simulink library "FInjLib"  (R2022b)
settings: Solver=VariableStepAuto  StartTime=0.0  StopTime=10.0  RelTol=1e-3
libraries: simulink x2, $bdroot x2
(part 1 of 2)
settings Model: Creator=flata  LastModifiedBy=JF
settings SolverCC: AlgebraicLoopSolver=TrustRegion
settings DebuggingCC: UnconnectedInputMsg=warning  UnconnectedOutputMsg=warning  UnconnectedLineMsg=warning  SFMachineParentedDataDiag=warning  ArithmeticOperatorsInVariantConditions=warning
settings ModelReferenceCC: EnableRefExpFcnMdlSchedulingChecks=on
settings SFSimCC: CustomCodeUndefinedFunction=UseInterfaceOnly
settings RTWCC: DLArmComputeVersion=19.05

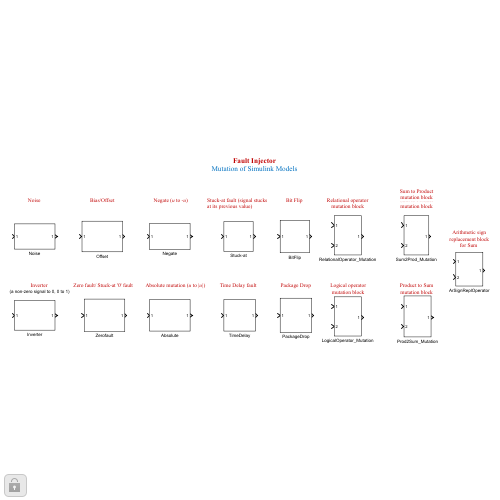
[thumbnail: Simulink's stored preview of the top-level diagram]
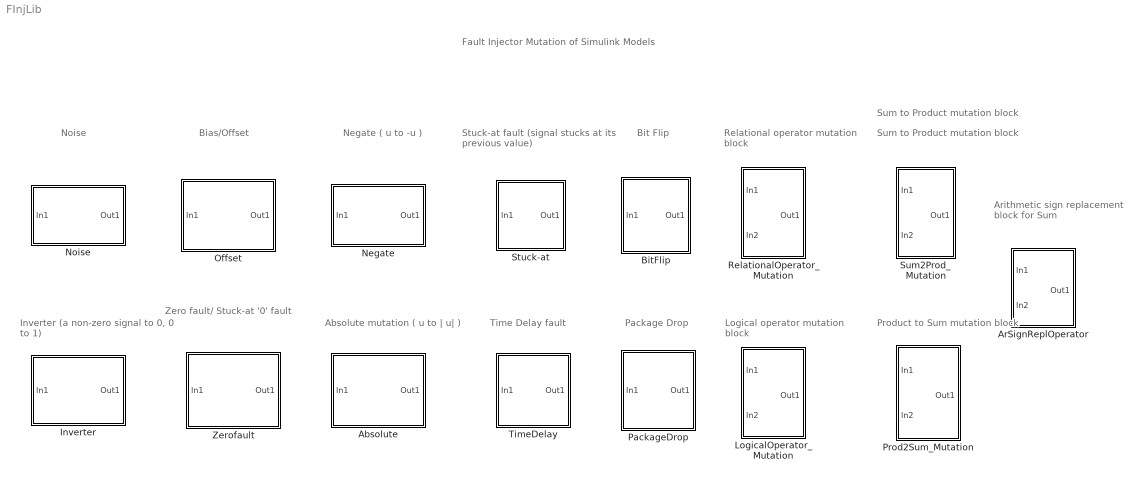
== system FInjLib ==
  note: Fault Injector
      | Mutation of Simulink Models
  note: Bias/Offset
  note: Noise
  note: Negate ( u to -u )
  note: Inverter
      | (a non-zero signal to 0, 0 to 1)
  note: Absolute mutation ( u to | u| )
  note: Zero fault/ Stuck-at '0' fault
  note: Stuck-at fault (signal stucks at its previous value)
  note: Time Delay fault
  note: Bit Flip
  note: Package Drop
  note: Relational operator mutation block
  note: Logical operator mutation block
  note: Sum to Product mutation block
  note: Product to Sum mutation block
  note: Arithmetic sign replacement block for Sum
  note: Sum to Product mutation block
  Absolute : Subsystem  mask(Absolue mutation block){FInjBlockNum=1, FIEnableflag=off, FaultOccurenceTime=0, FaultEffect=Infinite time, FaultDuration=1}
      mask prompts: FInjBlockNum "Name of the Fault Injector block"; FIEnableflag "Turn on fault injection"; FaultOccurenceTime "Enter the time of fault occurence (in seconds)"; FaultDuration "Enter the fault duration (in seconds)"
      mask help: This block makes a signal u to |u|.
      mask init:
      | a = Simulink.Mask.get(gcb);
      | Enable_signal = a.getParameter('FIEnableflag');
      | Fault_Occurence_Time = a.getParameter('FaultOccurenceTime');
      | Fault_Effect = a.getParameter('FaultEffect');
      | Fault_Duration = a.getParameter('FaultDuration');
      | 
      | value = Enable_signal.Value;
      | switch value
      |     case 'on'
      |     set_param('FInjLib/Absolute/Enable_flag', 'Value', '1');
      |     case 'off'
      |     set_param('FInjLib/Absolute/Enable_flag', 'Value', '0');
      | end
      | 
      | if Fault_Effect.Value == "Infinite time"
      |     Fault_Duration.Visible = 'off';
      | else
      |     Fault_Duration.Visible = 'on';
      | end
      | 
      | if Fault_Effect.Value == "Constant time"
      |     Fault_Duration.Prompt = "Enter the fault duration (in seconds)";
      | end
      | 
      | if Fault_Effect.Value == "Infinite time"
      |     set_param('FInjLib/Absolute/Faulttype','Value', '1');
      |     set_param('FInjLib/Absolute/Step', 'Time', Fault_Occurence_Time.Value);
      | else
      |     set_param('FInjLib/Absolute/Faulttype','Value', '2');
      |     set_param('FInjLib/Absolute/Pulse Generator', 'PhaseDelay', Fault_Occurence_Time.Value);
      |     set_param('FInjLib/Absolute/Pulse Generator', 'PulseWidth', Fault_Duration.Value);
      | end
      mask Help:
      | The block takes the following inputs:
      | - Name of the Fault Injector block ---- Feed a number as input
      | - Fault effect --- Constant time, Infinite time
      | - Fault duration --- if Fault effect is 'Constant time'
      | 
      | *For further information, see the file "README.m"
      mask TypeOptions FaultEffect: Infinite time | Constant time
      mask DialogControl Container3 Prompt: Fault Effect
  ArSignReplOperator : Subsystem  mask(Arithmetic Sign Replacement Block (for Sum)){FInjBlockNum=1, FIEnableflag=off, OperatorNum=2, FaultOccurenceTime=3, FaultEffect=Constant time, FaultDuration=5}
      mask prompts: FInjBlockNum "Name of the Fault Injector block"; FIEnableflag "Turn on fault injection"; OperatorNum "Enter the Operator Number from the above list"; FaultOccurenceTime "Enter the time of fault occurence (in seconds)"; FaultDuration "Enter the fault duration (in seconds)"
      mask help:
      | This block replaces the sign of the sum operator with the chosen one.
      |
      | Operator list:
      |
      | 1 : +-
      | 2 : --
      | 3 : ++
      | 4 : -+
      mask init:
      | a = Simulink.Mask.get(gcb);
      | Enable_signal = a.getParameter('FIEnableflag');
      | Fault_Occurence_Time = a.getParameter('FaultOccurenceTime');
      | Fault_Effect = a.getParameter('FaultEffect');
      | Fault_Duration = a.getParameter('FaultDuration');
      | Operator_Num = a.getParameter('OperatorNum');
      | 
      | value = Enable_signal.Value;
      | switch value
      |     case 'on'
      |     set_param('FInjLib/ArSignReplOperator/Enable_flag', 'Value', '1');
      |     case 'off'
      |     set_param('FInjLib/ArSignReplOperator/Enable_flag', 'Value', '0');
      | end
      | 
      | set_param('FInjLib/ArSignReplOperator/Operator Num', 'Value', Operator_Num.Value);
      | 
      | if Fault_Effect.Value == "Infinite time"
      |     Fault_Duration.Visible = 'off';
      | else
      |     Fault_Duration.Visible = 'on';
      | end
      | 
      | if Fault_Effect.Value == "Constant time"
      |     Fault_Duration.Prompt = "Enter the fault duration (in seconds)";
      | end
      | 
      | if Fault_Effect.Value == "Infinite time"
      |     set_param('FInjLib/ArSignReplOperator/Faulttype','Value', '1');
      |     set_param('FInjLib/ArSignReplOperator/Step', 'Time', Fault_Occurence_Time.Value);
      | else
      |     set_param('FInjLib/ArSignReplOperator/Faulttype','Value', '2');
      |     set_param('FInjLib/ArSignReplOperator/Pulse Generator', 'PhaseDelay', Fault_Occurence_Time.Value);
      |     set_param('FInjLib/ArSignReplOperator/Pulse Generator', 'PulseWidth', Fault_Duration.Value);
      | end
      mask Help:
      | The block takes the following inputs:
      | - Name of the Fault Injector block ---- Feed a number as input
      | - Operator Number -- Feed the operator number from the list of operators
      | - Fault effect --- Constant time, Infinite time
      | - Fault duration --- if Fault effect is 'Constant time'
      | 
      | *For further information, see the file "README.m"
      mask TypeOptions FaultEffect: Infinite time | Constant time
      mask DialogControl Container3 Prompt: Fault Effect
  BitFlip : Subsystem  mask(Bit Flips){FInjBlockNum=1, FIEnableflag=on, FaultOccurenceTime=0, FaultEffect=Infinite time, FaultDuration=0}
      mask prompts: FInjBlockNum "Name of the Fault Injector block"; FIEnableflag "Turn on fault injection"; FaultOccurenceTime "Enter the time of fault occurence (in seconds)"; FaultDuration "Enter the fault duration (in seconds)"
      mask help:
      | This block performs Bitwise NOT operation on the boolean signal.
      |  (The bits are inverted in the binary representation of the correct value).
      mask init:
      | a = Simulink.Mask.get(gcb);
      | Enable_signal = a.getParameter('FIEnableflag');
      | Fault_Occurence_Time = a.getParameter('FaultOccurenceTime');
      | Fault_Effect = a.getParameter('FaultEffect');
      | Fault_Duration = a.getParameter('FaultDuration');
      | 
      | value = Enable_signal.Value;
      | switch value
      |     case 'on'
      |     set_param('FInjLib/BitFlip/Enable_flag', 'Value', '1');
      |     case 'off'
      |     set_param('FInjLib/BitFlip/Enable_flag', 'Value', '0');
      | end
      | 
      | if Fault_Effect.Value == "Infinite time"
      |     Fault_Duration.Visible = 'off';
      | else
      |     Fault_Duration.Visible = 'on';
      | end
      | 
      | if Fault_Effect.Value == "Constant time"
      |     Fault_Duration.Prompt = "Enter the fault duration (in seconds)";
      | end
      | 
      | if Fault_Effect.Value == "Infinite time"
      |     set_param('FInjLib/BitFlip/Faulttype','Value', '1');
      |     set_param('FInjLib/BitFlip/Step', 'Time', Fault_Occurence_Time.Value);
      | else
      |     set_param('FInjLib/BitFlip/Faulttype','Value', '2');
      |     set_param('FInjLib/BitFlip/Pulse Generator', 'PhaseDelay', Fault_Occurence_Time.Value);
      |     set_param('FInjLib/BitFlip/Pulse Generator', 'PulseWidth', Fault_Duration.Value);
      | end
      mask Help:
      | The block takes the following inputs:
      | - Name of the Fault Injector block ---- Feed a number as input
      | - Fault effect --- Constant time, Infinite time
      | - Fault duration --- if Fault effect is 'Constant time'
      | 
      | *For further information, see the file "README.m"
      mask TypeOptions FaultEffect: Infinite time | Constant time
      mask DialogControl Container3 Prompt: Fault Effect
  Inverter : Subsystem  mask(Inverter){FInjBlockNum=1, FIEnableflag=off, FaultOccurenceTime=0, FaultEffect=Infinite time, FaultDuration=1}
      mask prompts: FInjBlockNum "Name of the Fault Injector block"; FIEnableflag "Turn on fault injection"; FaultOccurenceTime "Enter the time of fault occurence (in seconds)"; FaultDuration "Enter the fault duration (in seconds)"
      mask help: This block inverts a non-zero signal 'u' to 0; and 0 to 1.
      mask init:
      | a = Simulink.Mask.get(gcb);
      | Enable_signal = a.getParameter('FIEnableflag');
      | Fault_Occurence_Time = a.getParameter('FaultOccurenceTime');
      | Fault_Effect = a.getParameter('FaultEffect');
      | Fault_Duration = a.getParameter('FaultDuration');
      | 
      | value = Enable_signal.Value;
      | switch value
      |     case 'on'
      |     set_param('FInjLib/Inverter/Enable_flag', 'Value', '1');
      |     case 'off'
      |     set_param('FInjLib/Inverter/Enable_flag', 'Value', '0');
      | end
      | 
      | if Fault_Effect.Value == "Infinite time"
      |     Fault_Duration.Visible = 'off';
      | else
      |     Fault_Duration.Visible = 'on';
      | end
      | 
      | if Fault_Effect.Value == "Constant time"
      |     Fault_Duration.Prompt = "Enter the fault duration (in seconds)";
      | end
      | 
      | if Fault_Effect.Value == "Infinite time"
      |     set_param('FInjLib/Inverter/Faulttype','Value', '1');
      |     set_param('FInjLib/Inverter/Step', 'Time', Fault_Occurence_Time.Value);
      | else
      |     set_param('FInjLib/Inverter/Faulttype','Value', '2');
      |     set_param('FInjLib/Inverter/Pulse Generator', 'PhaseDelay', Fault_Occurence_Time.Value);
      |     set_param('FInjLib/Inverter/Pulse Generator', 'PulseWidth', Fault_Duration.Value);
      | end
      mask Help:
      | The block takes the following inputs:
      | - Name of the Fault Injector block ---- Feed a number as input
      | - Fault effect --- Constant time, Infinite time
      | - Fault duration --- if Fault effect is 'Constant time'
      | 
      | *For further information, see the file "README.m"
      mask TypeOptions FaultEffect: Infinite time | Constant time
      mask DialogControl Container3 Prompt: Fault Effect
  LogicalOperator_Mutation : Subsystem  mask(Logical Operator Replacement Block){FInjBlockNum=1, FIEnableflag=off, OperatorNum=4, FaultOccurenceTime=2, FaultEffect=Constant time, FaultDuration=3}
      mask prompts: FInjBlockNum "Name of the Fault Injector block"; FIEnableflag "Turn on fault injection"; OperatorNum "Enter the Operator Number from the above list"; FaultOccurenceTime "Enter the time of fault occurence (in seconds)"; FaultDuration "Enter the fault duration (in seconds)"
      mask help:
      | This block replaces the original logical operator with the chosen one.
      |
      | Operator list:
      |
      | 1 - AND
      | 2 - OR
      | 3 - NAND
      | 4 - NOR
      | 5 - XOR
      | 6 - NXOR
      mask init:
      | a = Simulink.Mask.get(gcb);
      | Enable_signal = a.getParameter('FIEnableflag');
      | Fault_Occurence_Time = a.getParameter('FaultOccurenceTime');
      | Fault_Effect = a.getParameter('FaultEffect');
      | Fault_Duration = a.getParameter('FaultDuration');
      | Operator_Num = a.getParameter('OperatorNum');
      | 
      | value = Enable_signal.Value;
      | switch value
      |     case 'on'
      |     set_param('FInjLib/LogicalOperator_Mutation/Enable_flag', 'Value', '1');
      |     case 'off'
      |     set_param('FInjLib/LogicalOperator_Mutation/Enable_flag', 'Value', '0');
      | end
      | 
      | set_param('FInjLib/LogicalOperator_Mutation/Operator Num', 'Value', Operator_Num.Value);
      | 
      | if Fault_Effect.Value == "Infinite time"
      |     Fault_Duration.Visible = 'off';
      | else
      |     Fault_Duration.Visible = 'on';
      | end
      | 
      | if Fault_Effect.Value == "Constant time"
      |     Fault_Duration.Prompt = "Enter the fault duration (in seconds)";
      | end
      | 
      | if Fault_Effect.Value == "Infinite time"
      |     set_param('FInjLib/LogicalOperator_Mutation/Faulttype','Value', '1');
      |     set_param('FInjLib/LogicalOperator_Mutation/Step', 'Time', Fault_Occurence_Time.Value);
      | else
      |     set_param('FInjLib/LogicalOperator_Mutation/Faulttype','Value', '2');
      |     set_param('FInjLib/LogicalOperator_Mutation/Pulse Generator', 'PhaseDelay', Fault_Occurence_Time.Value);
      |     set_param('FInjLib/LogicalOperator_Mutation/Pulse Generator', 'PulseWidth', Fault_Duration.Value);
      | end
      mask Help:
      | The block takes the following inputs:
      | - Name of the Fault Injector block ---- Feed a number as input
      | - Operator Number -- Feed the operator number from the list of operators
      | - Fault effect --- Constant time, Infinite time
      | - Fault duration --- if Fault effect is 'Constant time'
      | 
      | *For further information, see the file "README.m"
      mask TypeOptions FaultEffect: Infinite time | Constant time
      mask DialogControl Container3 Prompt: Fault Effect
  Negate : Subsystem  mask(Negate){FInjBlockNum=1, FIEnableflag=off, FaultOccurenceTime=4, FaultEffect=Infinite time, FaultDuration=1}
      mask prompts: FInjBlockNum "Name of the Fault Injector block"; FIEnableflag "Turn on fault injection"; FaultOccurenceTime "Enter the time of fault occurence (in seconds)"; FaultDuration "Enter the fault duration (in seconds)"
      mask help: This block makes a signal u to -u.
      mask init:
      | a = Simulink.Mask.get(gcb);
      | Enable_signal = a.getParameter('FIEnableflag');
      | Fault_Occurence_Time = a.getParameter('FaultOccurenceTime');
      | Fault_Effect = a.getParameter('FaultEffect');
      | Fault_Duration = a.getParameter('FaultDuration');
      | 
      | value = Enable_signal.Value;
      | switch value
      |     case 'on'
      |     set_param('FInjLib/Negate/Enable_flag', 'Value', '1');
      |     case 'off'
      |     set_param('FInjLib/Negate/Enable_flag', 'Value', '0');
      | end
      | 
      | if Fault_Effect.Value == "Infinite time"
      |     Fault_Duration.Visible = 'off';
      | else
      |     Fault_Duration.Visible = 'on';
      | end
      | 
      | if Fault_Effect.Value == "Constant time"
      |     Fault_Duration.Prompt = "Enter the fault duration (in seconds)";
      | end
      | 
      | if Fault_Effect.Value == "Infinite time"
      |     set_param('FInjLib/Negate/Faulttype','Value', '1');
      |     set_param('FInjLib/Negate/Step', 'Time', Fault_Occurence_Time.Value);
      | else
      |     set_param('FInjLib/Negate/Faulttype','Value', '2');
      |     set_param('FInjLib/Negate/Pulse Generator', 'PhaseDelay', Fault_Occurence_Time.Value);
      |     set_param('FInjLib/Negate/Pulse Generator', 'PulseWidth', Fault_Duration.Value);
      | end
      mask Help:
      | The block takes the following inputs:
      | - Name of the Fault Injector block ---- Feed a number as input
      | - Fault effect --- Constant time, Infinite time
      | - Fault duration --- if Fault effect is 'Constant time'
      | 
      | *For further information, see the file "README.m"
      mask TypeOptions FaultEffect: Infinite time | Constant time
      mask DialogControl Container3 Prompt: Fault Effect
  Noise : Subsystem  mask(Noise){FInjBlockNum=1, FIEnableflag=off, FaultValue=1, FaultOccurenceTime=2, FaultEffect=Constant time, FaultDuration=4}
      mask prompts: FInjBlockNum "Name of the Fault Injector block"; FIEnableflag "Turn on fault injection"; FaultValue "Fault value (Noise power)"; FaultOccurenceTime "Enter the time of fault occurence (in seconds)"; FaultDuration "Enter the fault duration (in seconds)"
      mask help: This block adds a band limited white noise to the input signal based on the specified fault value [noise power].
      mask init:
      | a = Simulink.Mask.get(gcb);
      | Enable_signal = a.getParameter('FIEnableflag');
      | Fault_value = a.getParameter('FaultValue');
      | Fault_Occurence_Time = a.getParameter('FaultOccurenceTime');
      | Fault_Effect = a.getParameter('FaultEffect');
      | Fault_Duration = a.getParameter('FaultDuration');
      | 
      | value = Enable_signal.Value;
      | switch value
      |     case 'on'
      |     set_param('FInjLib/Noise/Enable_flag', 'Value', '1');
      |     case 'off'
      |     set_param('FInjLib/Noise/Enable_flag', 'Value', '0');
      | end
      | Fault_value = a.getParameter('FaultValue');
      | set_param('FInjLib/Noise/Band-Limited White Noise', 'Cov', Fault_value.Value);
      | 
      | 
      | if Fault_Effect.Value == "Infinite time"
      |     Fault_Duration.Visible = 'off';
      | else
      |     Fault_Duration.Visible = 'on';
      | end
      | 
      | if Fault_Effect.Value == "Constant time"
      |     Fault_Duration.Prompt = "Enter the fault duration (in seconds)";
      | end
      | 
      | if Fault_Effect.Value == "Infinite time"
      |     set_param('FInjLib/Noise/Faulttype','Value', '1');
      |     set_param('FInjLib/Noise/Step', 'Time', Fault_Occurence_Time.Value);
      | else
      |     set_param('FInjLib/Noise/Faulttype','Value', '2');
      |     set_param('FInjLib/Noise/Pulse Generator', 'PhaseDelay', Fault_Occurence_Time.Value);
      |     set_param('FInjLib/Noise/Pulse Generator', 'PulseWidth', Fault_Duration.Value);
      | end
      mask Help:
      | The block takes the following inputs:
      | - Name of the Fault Injector block ---- Feed a number as input
      | - Fault value ---  the noise power
      | - Fault effect --- Constant time, Infinite time
      | - Fault duration --- if Fault effect is 'Constant time'
      | 
      | *For further information, see the file "README.m"
      mask TypeOptions FaultEffect: Infinite time | Constant time
      mask DialogControl Container3 Prompt: Fault Effect
  Offset : Subsystem  mask(Offset){FInjBlockNum=1, FIEnableflag=off, FaultValue=10, FaultOccurenceTime=2, FaultEffect=Constant time, FaultDuration=4}
      mask prompts: FInjBlockNum "Name of the Fault Injector block"; FIEnableflag "Turn on fault injection"; FaultValue "Fault value (Bias/Offset)"; FaultOccurenceTime "Enter the time of fault occurence (in seconds)"; FaultDuration "Enter the fault duration (in seconds)"
      mask help: This block adds a predefined +ve or -ve offset (bias) value to the input signal.
      mask init:
      | a = Simulink.Mask.get(gcb);
      | Enable_signal = a.getParameter('FIEnableflag');
      | Fault_value = a.getParameter('FaultValue');
      | Fault_Occurence_Time = a.getParameter('FaultOccurenceTime');
      | Fault_Effect = a.getParameter('FaultEffect');
      | Fault_Duration = a.getParameter('FaultDuration');
      | 
      | value = Enable_signal.Value;
      | switch value
      |     case 'on'
      |     set_param('FInjLib/Offset/Enable_flag', 'Value', '1');
      |     case 'off'
      |     set_param('FInjLib/Offset/Enable_flag', 'Value', '0');
      | end
      | Fault_value = a.getParameter('FaultValue');
      | set_param('FInjLib/Offset/Fault value', 'Value', Fault_value.Value);
      | 
      | if Fault_Effect.Value == "Infinite time"
      |     Fault_Duration.Visible = 'off';
      | else
      |     Fault_Duration.Visible = 'on';
      | end
      | 
      | if Fault_Effect.Value == "Constant time"
      |     Fault_Duration.Prompt = "Enter the fault duration (in seconds)";
      | end
      | 
      | if Fault_Effect.Value == "Infinite time"
      |     set_param('FInjLib/Offset/Faulttype','Value', '1');
      |     set_param('FInjLib/Offset/Step', 'Time', Fault_Occurence_Time.Value);
      | else
      |     set_param('FInjLib/Offset/Faulttype','Value', '2');
      |     set_param('FInjLib/Offset/Pulse Generator', 'PhaseDelay', Fault_Occurence_Time.Value);
      |     set_param('FInjLib/Offset/Pulse Generator', 'PulseWidth', Fault_Duration.Value);
      | end
      mask Help:
      | The block takes the following inputs:
      | - Name of the Fault Injector block ---- Feed a number as input
      | - Fault value ---  the bias/offset value
      | - Fault effect --- Constant time, Infinite time
      | - Fault duration --- if Fault effect is 'Constant time'
      | 
      | *For further information, see the file "README.m"
      mask TypeOptions FaultEffect: Infinite time | Constant time
      mask DialogControl Container3 Prompt: Fault Effect
  PackageDrop : Subsystem  mask(Package Drop){FInjBlockNum=1, FIEnableflag=on, FaultValue=0, FaultOccurenceTime=0, FaultEffect=Infinite time, FaultDuration=2}
      mask prompts: FInjBlockNum "Name of the Fault Injector block"; FIEnableflag "Turn on fault injection"; FaultValue "Fault value"; FaultOccurenceTime "Enter the time of fault occurence (in seconds)"; FaultDuration "Enter the fault duration (in seconds)"
      mask help:
      | This block replaces the input signal value by the specified fault value (mimicking a package drop in a network).
      | (The correct output is replaced by the specified fault value).
      mask init:
      | a = Simulink.Mask.get(gcb);
      | Enable_signal = a.getParameter('FIEnableflag');
      | Fault_value = a.getParameter('FaultValue');
      | Fault_Occurence_Time = a.getParameter('FaultOccurenceTime');
      | Fault_Effect = a.getParameter('FaultEffect');
      | Fault_Duration = a.getParameter('FaultDuration');
      | 
      | value = Enable_signal.Value;
      | switch value
      |     case 'on'
      |     set_param('FInjLib/PackageDrop/Enable_flag', 'Value', '1');
      |     case 'off'
      |     set_param('FInjLib/PackageDrop/Enable_flag', 'Value', '0');
      | end
      | Fault_value = a.getParameter('FaultValue');
      | set_param('FInjLib/PackageDrop/Fault value', 'Value', Fault_value.Value);
      | 
      | if Fault_Effect.Value == "Infinite time"
      |     Fault_Duration.Visible = 'off';
      | else
      |     Fault_Duration.Visible = 'on';
      | end
      | 
      | if Fault_Effect.Value == "Constant time"
      |     Fault_Duration.Prompt = "Enter the fault duration (in seconds)";
      | end
      | 
      | if Fault_Effect.Value == "Infinite time"
      |     set_param('FInjLib/PackageDrop/Faulttype','Value', '1');
      |     set_param('FInjLib/PackageDrop/Step', 'Time', Fault_Occurence_Time.Value);
      | else
      |     set_param('FInjLib/PackageDrop/Faulttype','Value', '2');
      |     set_param('FInjLib/PackageDrop/Pulse Generator', 'PhaseDelay', Fault_Occurence_Time.Value);
      |     set_param('FInjLib/PackageDrop/Pulse Generator', 'PulseWidth', Fault_Duration.Value);
      | end
      mask Help:
      | The block takes the following inputs:
      | - Name of the Fault Injector block ---- Feed a number as input
      | - Fault value ---  the input signal is replaced by this fault value
      | - Fault effect --- Constant time, Infinite time
      | - Fault duration --- if Fault effect is 'Constant time'
      | 
      | *For further information, see the file "README.m"
      mask TypeOptions FaultEffect: Infinite time | Constant time
      mask DialogControl Container3 Prompt: Fault Effect
  Prod2Sum_Mutation : Subsystem  mask(Product to Sum Mutation block){FInjBlockNum=1, FIEnableflag=off, FaultOccurenceTime=7, FaultEffect=Infinite time, FaultDuration=6}
      mask prompts: FInjBlockNum "Name of the Fault Injector block"; FIEnableflag "Turn on fault injection"; FaultOccurenceTime "Enter the time of fault occurence (in seconds)"; FaultDuration "Enter the fault duration (in seconds)"
      mask help: This block replaces multiplication operation with addition operation (between the two inputs for the specified time).
      mask init:
      | a = Simulink.Mask.get(gcb);
      | Enable_signal = a.getParameter('FIEnableflag');
      | Fault_Occurence_Time = a.getParameter('FaultOccurenceTime');
      | Fault_Effect = a.getParameter('FaultEffect');
      | Fault_Duration = a.getParameter('FaultDuration');
      | 
      | value = Enable_signal.Value;
      | switch value
      |     case 'on'
      |     set_param('FInjLib/Prod2Sum_Mutation/Enable_flag', 'Value', '1');
      |     case 'off'
      |     set_param('FInjLib/Prod2Sum_Mutation/Enable_flag', 'Value', '0');
      | end
      | 
      | if Fault_Effect.Value == "Infinite time"
      |     Fault_Duration.Visible = 'off';
      | else
      |     Fault_Duration.Visible = 'on';
      | end
      | 
      | if Fault_Effect.Value == "Constant time"
      |     Fault_Duration.Prompt = "Enter the fault duration (in seconds)";
      | end
      | 
      | if Fault_Effect.Value == "Infinite time"
      |     set_param('FInjLib/Prod2Sum_Mutation/Faulttype','Value', '1');
      |     set_param('FInjLib/Prod2Sum_Mutation/Step', 'Time', Fault_Occurence_Time.Value);
      | else
      |     set_param('FInjLib/Prod2Sum_Mutation/Faulttype','Value', '2');
      |     set_param('FInjLib/Prod2Sum_Mutation/Pulse Generator', 'PhaseDelay', Fault_Occurence_Time.Value);
      |     set_param('FInjLib/Prod2Sum_Mutation/Pulse Generator', 'PulseWidth', Fault_Duration.Value);
      | end
      mask Help:
      | The block takes the following inputs:
      | - Name of the Fault Injector block ---- Feed a number as input
      | - Fault effect --- Constant time, Infinite time
      | - Fault duration --- if Fault effect is 'Constant time'
      | 
      | *For further information, see the file "README.m"
      mask TypeOptions FaultEffect: Infinite time | Constant time
      mask DialogControl Container3 Prompt: Fault Effect
  RelationalOperator_Mutation : Subsystem  mask(Relational Operator Replacement Block){FInjBlockNum=1, FIEnableflag=off, OperatorNum=4, FaultOccurenceTime=2, FaultEffect=Constant time, FaultDuration=3}
      mask prompts: FInjBlockNum "Name of the Fault Injector block"; FIEnableflag "Turn on fault injection"; OperatorNum "Enter the Operator Number from the above list"; FaultOccurenceTime "Enter the time of fault occurence (in seconds)"; FaultDuration "Enter the fault duration (in seconds)"
      mask help:
      | This block replaces the original relational operator with the chosen one.
      |
      | Operator list:
      |
      | 1 - >
      | 2 - <
      | 3 - <=
      | 4 - >=
      | 5 - ==
      | 6 - ~=
      mask init:
      | a = Simulink.Mask.get(gcb);
      | Enable_signal = a.getParameter('FIEnableflag');
      | Fault_Occurence_Time = a.getParameter('FaultOccurenceTime');
      | Fault_Effect = a.getParameter('FaultEffect');
      | Fault_Duration = a.getParameter('FaultDuration');
      | Operator_Num = a.getParameter('OperatorNum');
      | 
      | value = Enable_signal.Value;
      | switch value
      |     case 'on'
      |     set_param('FInjLib/RelationalOperator_Mutation/Enable_flag', 'Value', '1');
      |     case 'off'
      |     set_param('FInjLib/RelationalOperator_Mutation/Enable_flag', 'Value', '0');
      | end
      | 
      | set_param('FInjLib/RelationalOperator_Mutation/Operator Num', 'Value', Operator_Num.Value);
      | 
      | if Fault_Effect.Value == "Infinite time"
      |     Fault_Duration.Visible = 'off';
      | else
      |     Fault_Duration.Visible = 'on';
      | end
      | 
      | if Fault_Effect.Value == "Constant time"
      |     Fault_Duration.Prompt = "Enter the fault duration (in seconds)";
      | end
      | 
      | if Fault_Effect.Value == "Infinite time"
      |     set_param('FInjLib/RelationalOperator_Mutation/Faulttype','Value', '1');
      |     set_param('FInjLib/RelationalOperator_Mutation/Step', 'Time', Fault_Occurence_Time.Value);
      | else
      |     set_param('FInjLib/RelationalOperator_Mutation/Faulttype','Value', '2');
      |     set_param('FInjLib/RelationalOperator_Mutation/Pulse Generator', 'PhaseDelay', Fault_Occurence_Time.Value);
      |     set_param('FInjLib/RelationalOperator_Mutation/Pulse Generator', 'PulseWidth', Fault_Duration.Value);
      | end
      mask Help:
      | The block takes the following inputs:
      | - Name of the Fault Injector block ---- Feed a number as input
      | - Operator Number -- Feed the operator number from the list of operators
      | - Fault effect --- Constant time, Infinite time
      | - Fault duration --- if Fault effect is 'Constant time'
      | 
      | *For further information, see the file "README.m"
      mask TypeOptions FaultEffect: Infinite time | Constant time
      mask DialogControl Container3 Prompt: Fault Effect
  Stuck-at : Subsystem  mask(Stuck-at fault){FInjBlockNum=1, FIEnableflag=on, FaultOccurenceTime=0, FaultEffect=Infinite time, FaultDuration=2}
      mask prompts: FInjBlockNum "Name of the Fault Injector block"; FIEnableflag "Turn on fault injection"; FaultOccurenceTime "Enter the time of fault occurence (in seconds)"; FaultEffect "Fault Effect"; FaultDuration "Enter the fault duration (in seconds)"
      mask help:
      | This block makes the input signal stuck at the value prior to fault occurence.
      | (The block output stays constant, preserving the latest correct value before the occurrence of the fault.)
      mask init:
      | a = Simulink.Mask.get(gcb);
      | Enable_signal = a.getParameter('FIEnableflag');
      | Fault_Occurence_Time = a.getParameter('FaultOccurenceTime');
      | Fault_Effect = a.getParameter('FaultEffect');
      | Fault_Duration = a.getParameter('FaultDuration');
      | 
      | value = Enable_signal.Value;
      | switch value
      |     case 'on'
      |     set_param('FInjLib/Stuck-at/Enable_flag', 'Value', '1');
      |     case 'off'
      |     set_param('FInjLib/Stuck-at/Enable_flag', 'Value', '0');
      | end
      | 
      | if Fault_Effect.Value == "Infinite time"
      |     Fault_Duration.Visible = 'off';
      | else
      |     Fault_Duration.Visible = 'on';
      | end
      | 
      | if Fault_Effect.Value == "Constant time"
      |     Fault_Duration.Prompt = "Enter the fault duration (in seconds)";
      | end
      | 
      | if Fault_Effect.Value == "Infinite time"
      |     set_param('FInjLib/Stuck-at/Faulttype','Value', '1');
      |     set_param('FInjLib/Stuck-at/Step', 'Time', Fault_Occurence_Time.Value);
      | else
      |     set_param('FInjLib/Stuck-at/Faulttype','Value', '2');
      |     set_param('FInjLib/Stuck-at/Pulse Generator', 'PhaseDelay', Fault_Occurence_Time.Value);
      |     set_param('FInjLib/Stuck-at/Pulse Generator', 'PulseWidth', Fault_Duration.Value);
      | end
      mask Help:
      | The block takes the following inputs:
      | - Name of the Fault Injector block ---- Feed a number as input
      | - Fault effect --- Constant time, Infinite time
      | - Fault duration --- if Fault effect is 'Constant time'
      | 
      | *For further information, see the file "README.m"
      mask TypeOptions FaultEffect: Infinite time | Constant time
  Sum2Prod_Mutation : Subsystem  mask(Sum to Product Mutation block){FInjBlockNum=1, FIEnableflag=off, FaultOccurenceTime=5, FaultEffect=Constant time, FaultDuration=3}
      mask prompts: FInjBlockNum "Name of the Fault Injector block"; FIEnableflag "Turn on fault injection"; FaultOccurenceTime "Enter the time of fault occurence (in seconds)"; FaultDuration "Enter the fault duration (in seconds)"
      mask help: This block replaces addition operation with multiplication operation (between the two inputs for the specified time).
      mask init:
      | a = Simulink.Mask.get(gcb);
      | Enable_signal = a.getParameter('FIEnableflag');
      | Fault_Occurence_Time = a.getParameter('FaultOccurenceTime');
      | Fault_Effect = a.getParameter('FaultEffect');
      | Fault_Duration = a.getParameter('FaultDuration');
      | 
      | value = Enable_signal.Value;
      | switch value
      |     case 'on'
      |     set_param('FInjLib/Sum2Prod_Mutation/Enable_flag', 'Value', '1');
      |     case 'off'
      |     set_param('FInjLib/Sum2Prod_Mutation/Enable_flag', 'Value', '0');
      | end
      | 
      | if Fault_Effect.Value == "Infinite time"
      |     Fault_Duration.Visible = 'off';
      | else
      |     Fault_Duration.Visible = 'on';
      | end
      | 
      | if Fault_Effect.Value == "Constant time"
      |     Fault_Duration.Prompt = "Enter the fault duration (in seconds)";
      | end
      | 
      | if Fault_Effect.Value == "Infinite time"
      |     set_param('FInjLib/Sum2Prod_Mutation/Faulttype','Value', '1');
      |     set_param('FInjLib/Sum2Prod_Mutation/Step', 'Time', Fault_Occurence_Time.Value);
      | else
      |     set_param('FInjLib/Sum2Prod_Mutation/Faulttype','Value', '2');
      |     set_param('FInjLib/Sum2Prod_Mutation/Pulse Generator', 'PhaseDelay', Fault_Occurence_Time.Value);
      |     set_param('FInjLib/Sum2Prod_Mutation/Pulse Generator', 'PulseWidth', Fault_Duration.Value);
      | end
      mask Help:
      | The block takes the following inputs:
      | - Name of the Fault Injector block ---- Feed a number as input
      | - Fault effect --- Constant time, Infinite time
      | - Fault duration --- if Fault effect is 'Constant time'
      | 
      | *For further information, see the file "README.m"
      mask TypeOptions FaultEffect: Infinite time | Constant time
      mask DialogControl Container3 Prompt: Fault Effect
  TimeDelay : Subsystem  mask(Time Delay){FInjBlockNum=1, FIEnableflag=off, FaultOccurenceTime=4, FaultEffect=Infinite time, FaultDuration=2}
      mask prompts: FInjBlockNum "Name of the Fault Injector block"; FIEnableflag "Turn on fault injection"; FaultOccurenceTime "Enter the time of fault occurence (in seconds)"; FaultEffect "Fault Effect"; FaultDuration "Enter the fault duration (in seconds)"
      mask help: This introduces a delay into the input signal. During the delay, the output stays constant, preserving the latest correct value before the occurrence of the fault.
      mask init:
      | a = Simulink.Mask.get(gcb);
      | Enable_signal = a.getParameter('FIEnableflag');
      | Fault_Occurence_Time = a.getParameter('FaultOccurenceTime');
      | Fault_Effect = a.getParameter('FaultEffect');
      | Fault_Duration = a.getParameter('FaultDuration');
      | 
      | value = Enable_signal.Value;
      | switch value
      |     case 'on'
      |     set_param('FInjLib/TimeDelay/Enable_flag', 'Value', '1');
      |     case 'off'
      |     set_param('FInjLib/TimeDelay/Enable_flag', 'Value', '0');
      | end
      | 
      | if Fault_Effect.Value == "Infinite time"
      |     Fault_Duration.Visible = 'off';
      | else
      |     Fault_Duration.Visible = 'on';
      | end
      | 
      | if Fault_Effect.Value == "Constant time"
      |     Fault_Duration.Prompt = "Enter the fault duration (in seconds)";
      | end
      | 
      | if Fault_Effect.Value == "Infinite time"
      |     set_param('FInjLib/TimeDelay/Faulttype','Value', '1');
      |     set_param('FInjLib/TimeDelay/Step', 'Time', Fault_Occurence_Time.Value);
      | else
      |     set_param('FInjLib/TimeDelay/Faulttype','Value', '2');
      |     set_param('FInjLib/TimeDelay/Pulse Generator', 'PhaseDelay', Fault_Occurence_Time.Value);
      |     set_param('FInjLib/TimeDelay/Pulse Generator', 'PulseWidth', Fault_Duration.Value);
      |     step_new = str2num(Fault_Occurence_Time.Value) +  str2num(Fault_Duration.Value);
      |     set_param('FInjLib/TimeDelay/Step1', 'Time', num2str(step_new));
      |     set_param('FInjLib/TimeDelay/Transport Delay', 'DelayTime', Fault_Duration.Value);
      |     
      | end
      mask Help:
      | The block takes the following inputs:
      | - Name of the Fault Injector block ---- Feed a number as input
      | - Fault effect --- Constant time, Infinite time
      | - Fault duration --- if Fault effect is 'Constant time'
      | 
      | *For further information, see the file "README.m"
      mask TypeOptions FaultEffect: Infinite time | Constant time
  Zerofault : Subsystem  mask(Zero fault (Stuck-at '0')){FInjBlockNum=1, FIEnableflag=off, FaultOccurenceTime=2, FaultEffect=Constant time, FaultDuration=4}
      mask prompts: FInjBlockNum "Name of the Fault Injector block"; FIEnableflag "Turn on fault injection"; FaultOccurenceTime "Enter the time of fault occurence (in seconds)"; FaultDuration "Enter the fault duration (in seconds)"
      mask help: This block makes the signal value '0' for the specified time.
      mask init:
      | a = Simulink.Mask.get(gcb);
      | Enable_signal = a.getParameter('FIEnableflag');
      | Fault_Occurence_Time = a.getParameter('FaultOccurenceTime');
      | Fault_Effect = a.getParameter('FaultEffect');
      | Fault_Duration = a.getParameter('FaultDuration');
      | 
      | value = Enable_signal.Value;
      | switch value
      |     case 'on'
      |     set_param('FInjLib/Zerofault/Enable_flag', 'Value', '1');
      |     case 'off'
      |     set_param('FInjLib/Zerofault/Enable_flag', 'Value', '0');
      | end
      | 
      | if Fault_Effect.Value == "Infinite time"
      |     Fault_Duration.Visible = 'off';
      | else
      |     Fault_Duration.Visible = 'on';
      | end
      | 
      | if Fault_Effect.Value == "Constant time"
      |     Fault_Duration.Prompt = "Enter the fault duration (in seconds)";
      | end
      | 
      | if Fault_Effect.Value == "Infinite time"
      |     set_param('FInjLib/Zerofault/Faulttype','Value', '1');
      |     set_param('FInjLib/Zerofault/Step', 'Time', Fault_Occurence_Time.Value);
      | else
      |     set_param('FInjLib/Zerofault/Faulttype','Value', '2');
      |     set_param('FInjLib/Zerofault/Pulse Generator', 'PhaseDelay', Fault_Occurence_Time.Value);
      |     set_param('FInjLib/Zerofault/Pulse Generator', 'PulseWidth', Fault_Duration.Value);
      | end
      mask Help:
      | The block takes the following inputs:
      | - Name of the Fault Injector block ---- Feed a number as input
      | - Fault effect --- Constant time, Infinite time
      | - Fault duration --- if Fault effect is 'Constant time'
      | 
      | *For further information, see the file "README.m"
      mask TypeOptions FaultEffect: Infinite time | Constant time
      mask DialogControl Container3 Prompt: Fault Effect

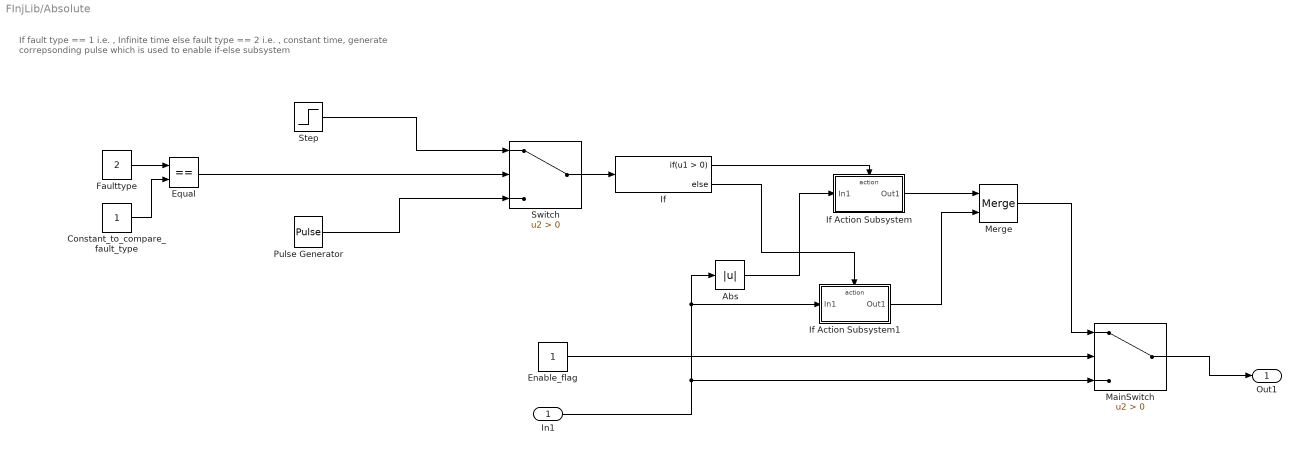
== system FInjLib/Absolute ==
  note: If fault type == 1 i.e. , Infinite time
      | else fault type == 2 i.e. , constant time,
      | generate correpsonding pulse which is used to enable if-else subsystem
  In1 : Inport
  Abs : Abs  SaturateOnIntegerOverflow=off
  Constant_to_compare_fault_type : Constant
  Enable_flag : Constant
  Equal : RelationalOperator  Operator===  OutDataTypeStr=boolean  RndMeth=Simplest  InputSameDT=off
  Faulttype : Constant  Value=2
  If : If
  If Action Subsystem : Subsystem  TreatAsAtomicUnit=on
  If Action Subsystem1 : Subsystem  TreatAsAtomicUnit=on
  MainSwitch : Switch  Criteria=u2 > Threshold  SaturateOnIntegerOverflow=off  InputSameDT=off
  Merge : Merge
  Pulse Generator : DiscretePulseGenerator  Period=500  PulseWidth=3  PhaseDelay=2
  Step : Step  Time=0  SampleTime=0
  Switch : Switch  Criteria=u2 > Threshold  SaturateOnIntegerOverflow=off  InputSameDT=off
  Out1 : Outport  VectorParamsAs1DForOutWhenUnconnected=off
  wires:
  MainSwitch/1 -> Out1/1
  Merge/1 -> MainSwitch/1
  Enable_flag/1 -> MainSwitch/2
  If Action Subsystem1/1(Out1) -> Merge/2
  Switch/1 -> If/1
  Abs/1 -> If Action Subsystem/1(In1)
  If/2 -> If Action Subsystem1/Action
  In1/1 -> MainSwitch/3, Abs/1, If Action Subsystem1/1(In1)
  If Action Subsystem/1(Out1) -> Merge/1
  If/1 -> If Action Subsystem/Action
  Step/1 -> Switch/1
  Faulttype/1 -> Equal/1
  Equal/1 -> Switch/2
  Pulse Generator/1 -> Switch/3
  Constant_to_compare_fault_type/1 -> Equal/2

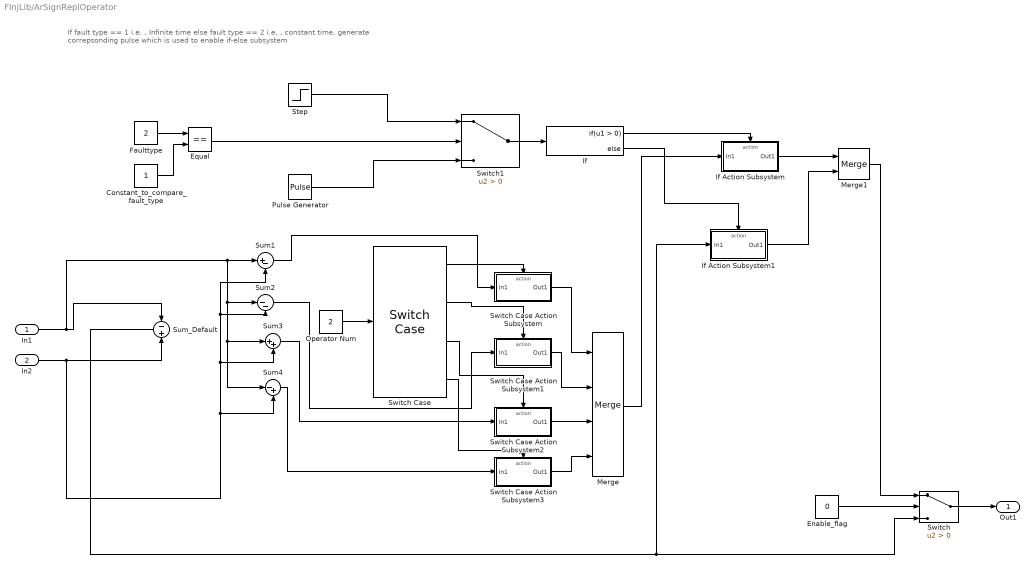
== system FInjLib/ArSignReplOperator ==
  note: If fault type == 1 i.e. , Infinite time
      | else fault type == 2 i.e. , constant time,
      | generate correpsonding pulse which is used to enable if-else subsystem
  In1 : Inport
  In2 : Inport  Port=2
  Constant_to_compare_fault_type : Constant
  Enable_flag : Constant  Value=0
  Equal : RelationalOperator  Operator===  OutDataTypeStr=boolean  RndMeth=Simplest  InputSameDT=off
  Faulttype : Constant  Value=2
  If : If
  If Action Subsystem : Subsystem  TreatAsAtomicUnit=on
  If Action Subsystem1 : Subsystem  TreatAsAtomicUnit=on
  Merge : Merge  Inputs=4
  Merge1 : Merge
  Operator Num : Constant  Value=2
  Pulse Generator : DiscretePulseGenerator  Period=500  PulseWidth=5  PhaseDelay=3
  Step : Step  Time=2  SampleTime=0
  Sum1 : Sum  Inputs=|+-
  Sum2 : Sum  Inputs=|--
  Sum3 : Sum  Inputs=|++
  Sum4 : Sum  Inputs=|-+
  Sum_Default : Sum  Inputs=-+
  Switch : Switch  Criteria=u2 > Threshold  SaturateOnIntegerOverflow=off  InputSameDT=off
  Switch Case : SwitchCase  CaseConditions={1,2,3,4}  ShowDefaultCase=off
  Switch Case Action Subsystem : Subsystem  TreatAsAtomicUnit=on
  Switch Case Action Subsystem1 : Subsystem  TreatAsAtomicUnit=on
  Switch Case Action Subsystem2 : Subsystem  TreatAsAtomicUnit=on
  Switch Case Action Subsystem3 : Subsystem  TreatAsAtomicUnit=on
  Switch1 : Switch  Criteria=u2 > Threshold  SaturateOnIntegerOverflow=off  InputSameDT=off
  Out1 : Outport  VectorParamsAs1DForOutWhenUnconnected=off
  wires:
  Switch/1 -> Out1/1
  Sum1/1 -> Switch Case Action Subsystem/1(In1)
  Merge1/1 -> Switch/1
  Switch Case Action Subsystem1/1(Out1) -> Merge/2
  Equal/1 -> Switch1/2
  Switch Case/4 -> Switch Case Action Subsystem3/Action
  Operator Num/1 -> Switch Case/1
  Pulse Generator/1 -> Switch1/3
  Switch Case/2 -> Switch Case Action Subsystem1/Action
  Sum2/1 -> Switch Case Action Subsystem1/1(In1)
  Faulttype/1 -> Equal/1
  Switch Case Action Subsystem2/1(Out1) -> Merge/3
  Constant_to_compare_fault_type/1 -> Equal/2
  Step/1 -> Switch1/1
  Switch1/1 -> If/1
  Switch Case Action Subsystem3/1(Out1) -> Merge/4
  Merge/1 -> If Action Subsystem/1(In1)
  If/1 -> If Action Subsystem/Action
  Switch Case Action Subsystem/1(Out1) -> Merge/1
  Sum4/1 -> Switch Case Action Subsystem3/1(In1)
  Sum3/1 -> Switch Case Action Subsystem2/1(In1)
  Switch Case/3 -> Switch Case Action Subsystem2/Action
  If/2 -> If Action Subsystem1/Action
  Sum_Default/1 -> Switch/3, If Action Subsystem1/1(In1)
  In2/1 -> Sum_Default/2, Sum2/2, Sum1/2, Sum3/2, Sum4/2
  Switch Case/1 -> Switch Case Action Subsystem/Action
  Enable_flag/1 -> Switch/2
  In1/1 -> Sum1/1, Sum4/1, Sum3/1, Sum2/1, Sum_Default/1
  If Action Subsystem1/1(Out1) -> Merge1/2
  If Action Subsystem/1(Out1) -> Merge1/1

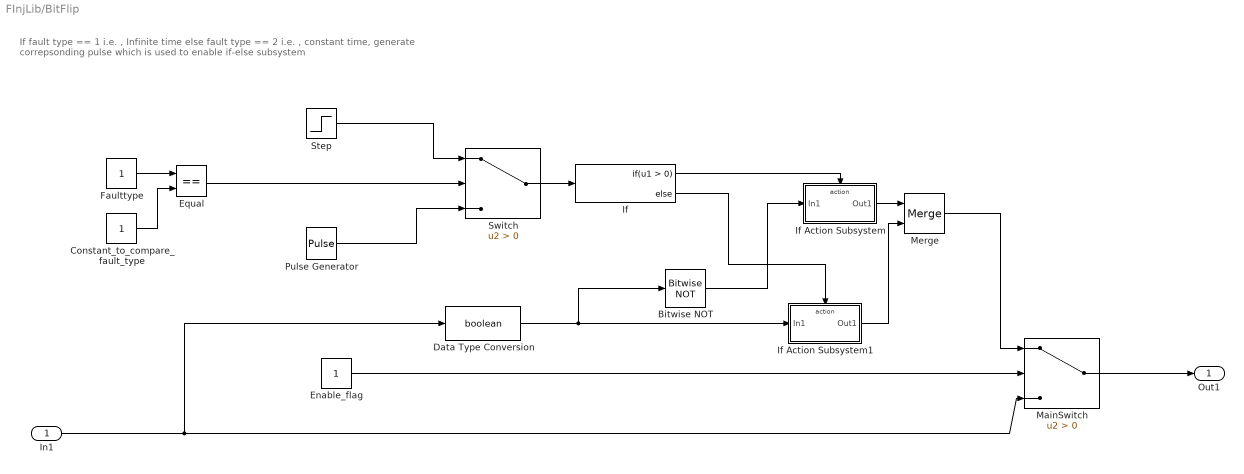
== system FInjLib/BitFlip ==
  note: If fault type == 1 i.e. , Infinite time
      | else fault type == 2 i.e. , constant time,
      | generate correpsonding pulse which is used to enable if-else subsystem
  In1 : Inport
  Bitwise NOT : simulink/Logic and Bit Operations/Bitwise Operator  logicop=NOT  UseBitMask=off  BitMask=bin2dec('11011001')  BitMaskRealWorld=Stored Integer
  Constant_to_compare_fault_type : Constant
  Data Type Conversion : DataTypeConversion  OutDataTypeStr=boolean  SaturateOnIntegerOverflow=off  RndMeth=Floor
  Enable_flag : Constant
  Equal : RelationalOperator  Operator===  OutDataTypeStr=boolean  RndMeth=Simplest  InputSameDT=off
  Faulttype : Constant
  If : If
  If Action Subsystem : Subsystem  TreatAsAtomicUnit=on
  If Action Subsystem1 : Subsystem  TreatAsAtomicUnit=on
  MainSwitch : Switch  Criteria=u2 > Threshold  SaturateOnIntegerOverflow=off  InputSameDT=off
  Merge : Merge
  Pulse Generator : DiscretePulseGenerator  Period=500  PulseWidth=5  PhaseDelay=3
  Step : Step  Time=0  SampleTime=0
  Switch : Switch  Criteria=u2 > Threshold  SaturateOnIntegerOverflow=off  InputSameDT=off
  Out1 : Outport  VectorParamsAs1DForOutWhenUnconnected=off
  wires:
  If/2 -> If Action Subsystem1/Action
  Constant_to_compare_fault_type/1 -> Equal/2
  Data Type Conversion/1 -> Bitwise NOT/1, If Action Subsystem1/1(In1)
  Switch/1 -> If/1
  If Action Subsystem/1(Out1) -> Merge/1
  Merge/1 -> MainSwitch/1
  If/1 -> If Action Subsystem/Action
  Equal/1 -> Switch/2
  Enable_flag/1 -> MainSwitch/2
  Faulttype/1 -> Equal/1
  Pulse Generator/1 -> Switch/3
  MainSwitch/1 -> Out1/1
  Bitwise NOT/1 -> If Action Subsystem/1(In1)
  If Action Subsystem1/1(Out1) -> Merge/2
  In1/1 -> Data Type Conversion/1, MainSwitch/3
  Step/1 -> Switch/1

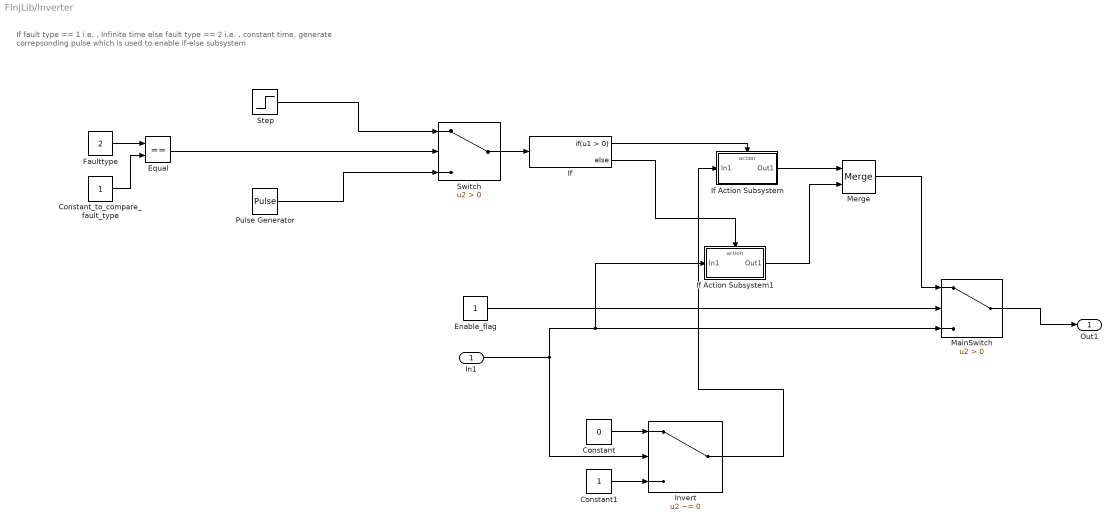
== system FInjLib/Inverter ==
  note: If fault type == 1 i.e. , Infinite time
      | else fault type == 2 i.e. , constant time,
      | generate correpsonding pulse which is used to enable if-else subsystem
  In1 : Inport
  Constant : Constant  Value=0
  Constant1 : Constant
  Constant_to_compare_fault_type : Constant
  Enable_flag : Constant
  Equal : RelationalOperator  Operator===  OutDataTypeStr=boolean  RndMeth=Simplest  InputSameDT=off
  Faulttype : Constant  Value=2
  If : If
  If Action Subsystem : Subsystem  TreatAsAtomicUnit=on
  If Action Subsystem1 : Subsystem  TreatAsAtomicUnit=on
  Invert : Switch  Criteria=u2 ~= 0  SaturateOnIntegerOverflow=off  InputSameDT=off
  MainSwitch : Switch  Criteria=u2 > Threshold  SaturateOnIntegerOverflow=off  InputSameDT=off
  Merge : Merge
  Pulse Generator : DiscretePulseGenerator  Period=500  PulseWidth=3  PhaseDelay=2
  Step : Step  Time=0  SampleTime=0
  Switch : Switch  Criteria=u2 > Threshold  SaturateOnIntegerOverflow=off  InputSameDT=off
  Out1 : Outport  VectorParamsAs1DForOutWhenUnconnected=off
  wires:
  Faulttype/1 -> Equal/1
  MainSwitch/1 -> Out1/1
  If/2 -> If Action Subsystem1/Action
  If/1 -> If Action Subsystem/Action
  Step/1 -> Switch/1
  If Action Subsystem1/1(Out1) -> Merge/2
  Invert/1 -> If Action Subsystem/1(In1)
  In1/1 -> Invert/2, MainSwitch/3, If Action Subsystem1/1(In1)
  Merge/1 -> MainSwitch/1
  Constant_to_compare_fault_type/1 -> Equal/2
  Switch/1 -> If/1
  Enable_flag/1 -> MainSwitch/2
  Equal/1 -> Switch/2
  If Action Subsystem/1(Out1) -> Merge/1
  Pulse Generator/1 -> Switch/3
  Constant/1 -> Invert/1
  Constant1/1 -> Invert/3

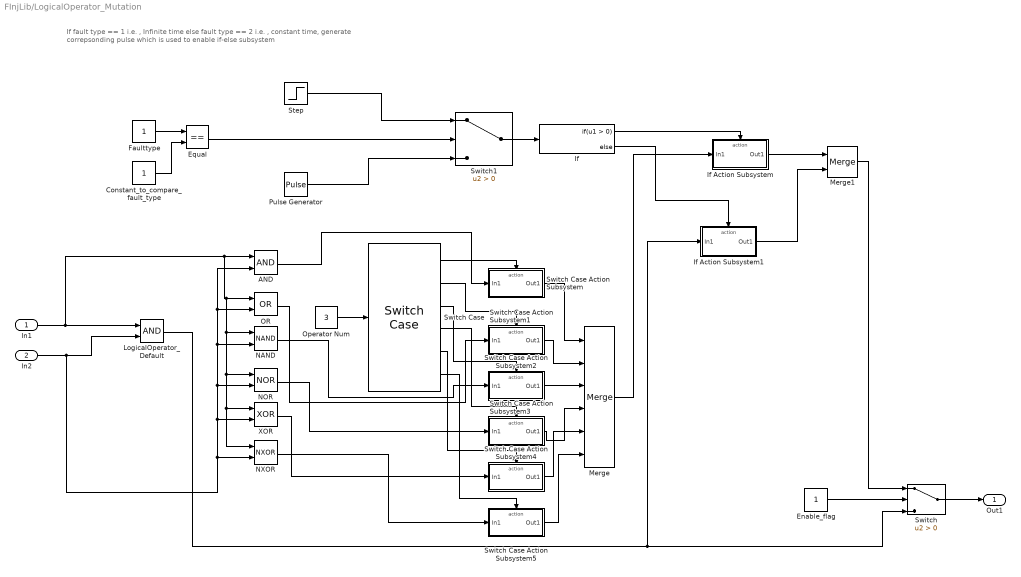
== system FInjLib/LogicalOperator_Mutation ==
  note: If fault type == 1 i.e. , Infinite time
      | else fault type == 2 i.e. , constant time,
      | generate correpsonding pulse which is used to enable if-else subsystem
  In1 : Inport
  In2 : Inport  Port=2
  AND : Logic  AllPortsSameDT=off  OutDataTypeStr=boolean
  Constant_to_compare_fault_type : Constant
  Enable_flag : Constant
  Equal : RelationalOperator  Operator===  OutDataTypeStr=boolean  RndMeth=Simplest  InputSameDT=off
  Faulttype : Constant
  If : If
  If Action Subsystem : Subsystem  TreatAsAtomicUnit=on
  If Action Subsystem1 : Subsystem  TreatAsAtomicUnit=on
  LogicalOperator_Default : Logic  AllPortsSameDT=off  OutDataTypeStr=boolean
  Merge : Merge  Inputs=6
  Merge1 : Merge
  NAND : Logic  Operator=NAND  AllPortsSameDT=off  OutDataTypeStr=boolean
  NOR : Logic  Operator=NOR  AllPortsSameDT=off  OutDataTypeStr=boolean
  NXOR : Logic  Operator=NXOR  AllPortsSameDT=off  OutDataTypeStr=boolean
  OR : Logic  Operator=OR  AllPortsSameDT=off  OutDataTypeStr=boolean
  Operator Num : Constant  Value=3
  Pulse Generator : DiscretePulseGenerator  Period=500  PulseWidth=4  PhaseDelay=3
  Step : Step  Time=3  SampleTime=0
  Switch : Switch  Criteria=u2 > Threshold  SaturateOnIntegerOverflow=off  InputSameDT=off
  Switch Case : SwitchCase  CaseConditions={1,2,3,4,5,6}  ShowDefaultCase=off
  Switch Case Action Subsystem : Subsystem  TreatAsAtomicUnit=on
  Switch Case Action Subsystem1 : Subsystem  TreatAsAtomicUnit=on
  Switch Case Action Subsystem2 : Subsystem  TreatAsAtomicUnit=on
  Switch Case Action Subsystem3 : Subsystem  TreatAsAtomicUnit=on
  Switch Case Action Subsystem4 : Subsystem  TreatAsAtomicUnit=on
  Switch Case Action Subsystem5 : Subsystem  TreatAsAtomicUnit=on
  Switch1 : Switch  Criteria=u2 > Threshold  SaturateOnIntegerOverflow=off  InputSameDT=off
  XOR : Logic  Operator=XOR  AllPortsSameDT=off  OutDataTypeStr=boolean
  Out1 : Outport  VectorParamsAs1DForOutWhenUnconnected=off
  wires:
  Switch Case Action Subsystem3/1(Out1) -> Merge/4
  Switch1/1 -> If/1
  Switch Case/4 -> Switch Case Action Subsystem3/Action
  AND/1 -> Switch Case Action Subsystem/1(In1)
  Switch Case/5 -> Switch Case Action Subsystem4/Action
  Switch Case Action Subsystem/1(Out1) -> Merge/1
  OR/1 -> Switch Case Action Subsystem1/1(In1)
  Enable_flag/1 -> Switch/2
  Switch Case Action Subsystem5/1(Out1) -> Merge/6
  If Action Subsystem/1(Out1) -> Merge1/1
  Switch/1 -> Out1/1
  Switch Case Action Subsystem2/1(Out1) -> Merge/3
  In2/1 -> LogicalOperator_Default/2, NAND/2, OR/2, AND/2, NOR/2, XOR/2, NXOR/2
  NOR/1 -> Switch Case Action Subsystem3/1(In1)
  Switch Case Action Subsystem4/1(Out1) -> Merge/5
  NAND/1 -> Switch Case Action Subsystem2/1(In1)
  Faulttype/1 -> Equal/1
  If/1 -> If Action Subsystem/Action
  LogicalOperator_Default/1 -> Switch/3, If Action Subsystem1/1(In1)
  XOR/1 -> Switch Case Action Subsystem4/1(In1)
  Merge/1 -> If Action Subsystem/1(In1)
  Operator Num/1 -> Switch Case/1
  Switch Case/6 -> Switch Case Action Subsystem5/Action
  Switch Case Action Subsystem1/1(Out1) -> Merge/2
  Switch Case/3 -> Switch Case Action Subsystem2/Action
  Equal/1 -> Switch1/2
  If Action Subsystem1/1(Out1) -> Merge1/2
  Constant_to_compare_fault_type/1 -> Equal/2
  Merge1/1 -> Switch/1
  If/2 -> If Action Subsystem1/Action
  In1/1 -> LogicalOperator_Default/1, AND/1, OR/1, NAND/1, NOR/1, NXOR/1, XOR/1
  Switch Case/1 -> Switch Case Action Subsystem/Action
  Pulse Generator/1 -> Switch1/3
  NXOR/1 -> Switch Case Action Subsystem5/1(In1)
  Switch Case/2 -> Switch Case Action Subsystem1/Action
  Step/1 -> Switch1/1
